simulink model "system_IIR_bank_decoder_AWGN"  (Simulink 8.3)
settings: Solver=ode45  StartTime=0.0  StopTime=10  RelTol=1e-3
undefined symbols (not defined in the file or in its folder): dfilt, fdesignblkfcn, gcbh
libraries: dsparch4 x7, commutil2 x2, commchan3 x1
settings Model: Creator=Vasilis  LastModifiedBy=Vasilis
settings DataIOCC: SignalLoggingSaveFormat=Dataset
settings DebuggingCC: UnderspecifiedInitializationDetection=Simplified  StateNameClashWarn=none
settings GRTTargetCC: CombineOutputUpdateFcns=on  GRTInterface=off

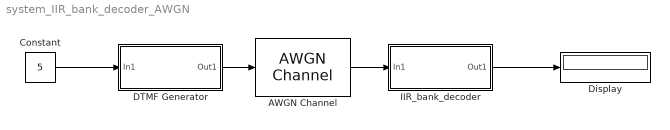
== system system_IIR_bank_decoder_AWGN ==
  AWGN Channel : commchan3/AWGN Channel  InputProcessing=Columns as channels (frame based)  seed=67  noiseMode="Signal to noise ratio  (SNR)"  EbNodB=10  EsNodB=10  SNRdB=0  bitsPerSym=1  Ps=1  Tsym=1  variance=1
  Constant : Constant  Value=5
  DTMF Generator : Subsystem
  Display : Display
  IIR_bank_decoder : Subsystem
  wires:
  DTMF Generator/1(Out1) -> AWGN Channel/1
  IIR_bank_decoder/1(Out1) -> Display/1
  Constant/1 -> DTMF Generator/1(In1)
  AWGN Channel/1 -> IIR_bank_decoder/1(In1)

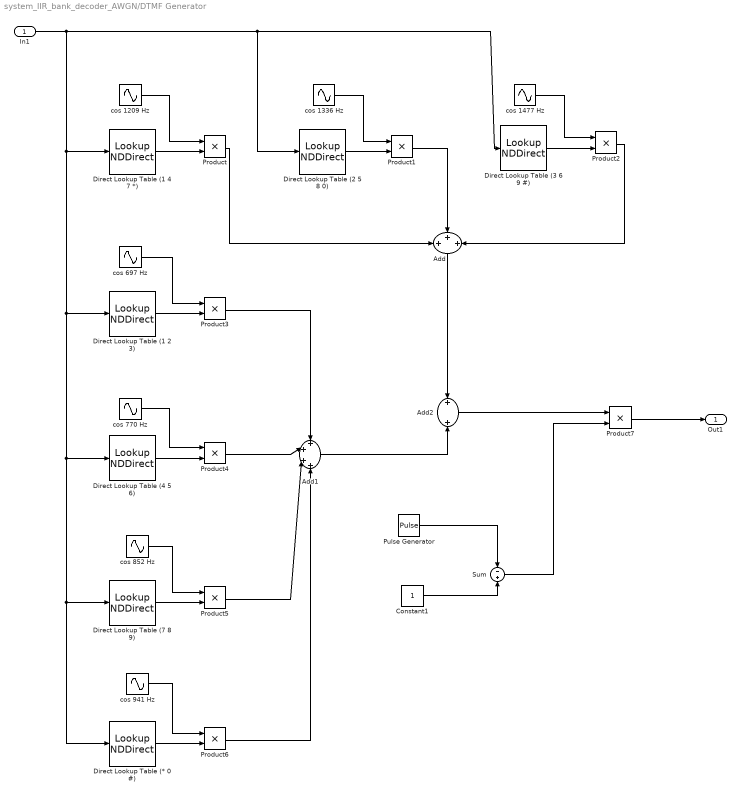
== system system_IIR_bank_decoder_AWGN/DTMF Generator ==
  In1 : Inport
  Add : Sum  Inputs=+++
  Add1 : Sum  Inputs=++++
  Add2 : Sum
  Constant1 : Constant
  Direct Lookup Table (* 0 #) : LookupNDDirect  NumberOfTableDimensions=1  Table=[1 0 0 0 0 0 0 0 0 0 1 1]
  Direct Lookup Table (1 2 3) : LookupNDDirect  NumberOfTableDimensions=1  Table=[0 1 1 1 0 0 0 0 0 0 0 0]
  Direct Lookup Table (1 4 7 *) : LookupNDDirect  NumberOfTableDimensions=1  Table=[0 1 0 0 1 0 0 1 0 0 1 0]
  Direct Lookup Table (2 5 8 0) : LookupNDDirect  NumberOfTableDimensions=1  Table=[1 0 1 0 0 1 0 0 1 0 0 0]
  Direct Lookup Table (3 6 9 #) : LookupNDDirect  NumberOfTableDimensions=1  Table=[0 0 0 1 0 0 1 0 0 1 0 1]
  Direct Lookup Table (4 5 6) : LookupNDDirect  NumberOfTableDimensions=1  Table=[0 0 0 0 1 1 1 0 0 0 0 0]
  Direct Lookup Table (7 8 9) : LookupNDDirect  NumberOfTableDimensions=1  Table=[0 0 0 0 0 0 0 1 1 1 0 0]
  Product{,1..7} (8 alike) : Product  RndMeth=Zero
  Pulse Generator : DiscretePulseGenerator  Period=480  PulseWidth=160  PhaseDelay=320  SampleTime=1/8000
  Sum : Sum  Inputs=-|+
  cos 1209 Hz : Sin  Frequency=7596  Phase=pi/2  SampleTime=1/8000
  cos 1336 Hz : Sin  Frequency=8394  Phase=pi/2  SampleTime=1/8000
  cos 1477 Hz : Sin  Frequency=9280  Phase=pi/2  SampleTime=1/8000
  cos 697 Hz : Sin  Frequency=4379  Phase=pi/2  SampleTime=1/8000
  cos 770 Hz : Sin  Frequency=4838  Phase=pi/2  SampleTime=1/8000
  cos 852 Hz : Sin  Frequency=5353  Phase=pi/2  SampleTime=1/8000
  cos 941 Hz : Sin  Frequency=5912  Phase=pi/2  SampleTime=1/8000
  Out1 : Outport
  wires:
  Direct Lookup Table (1 4 7 *)/1 -> Product/2
  In1/1 -> Direct Lookup Table (2 5 8 0)/1, Direct Lookup Table (3 6 9 #)/1, Direct Lookup Table (1 4 7 *)/1, Direct Lookup Table (1 2 3)/1, Direct Lookup Table (4 5 6)/1, Direct Lookup Table (7 8 9)/1, Direct Lookup Table (* 0 #)/1
  cos 1336 Hz/1 -> Product1/1
  Direct Lookup Table (2 5 8 0)/1 -> Product1/2
  cos 1477 Hz/1 -> Product2/1
  Direct Lookup Table (3 6 9 #)/1 -> Product2/2
  cos 697 Hz/1 -> Product3/1
  Direct Lookup Table (1 2 3)/1 -> Product3/2
  cos 770 Hz/1 -> Product4/1
  Direct Lookup Table (4 5 6)/1 -> Product4/2
  cos 852 Hz/1 -> Product5/1
  Direct Lookup Table (7 8 9)/1 -> Product5/2
  Product2/1 -> Add/3
  Product1/1 -> Add/2
  Product/1 -> Add/1
  Product3/1 -> Add1/1
  Product5/1 -> Add1/3
  Product4/1 -> Add1/2
  Add1/1 -> Add2/2
  Add/1 -> Add2/1
  cos 941 Hz/1 -> Product6/1
  Direct Lookup Table (* 0 #)/1 -> Product6/2
  Product6/1 -> Add1/4
  cos 1209 Hz/1 -> Product/1
  Constant1/1 -> Sum/2
  Pulse Generator/1 -> Sum/1
  Product7/1 -> Out1/1
  Add2/1 -> Product7/1
  Sum/1 -> Product7/2

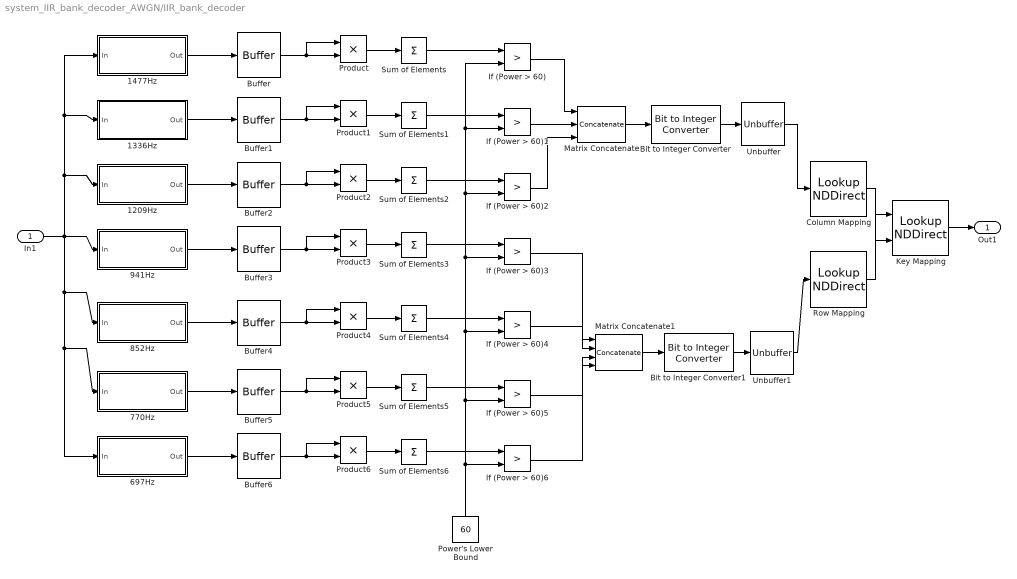
== system system_IIR_bank_decoder_AWGN/IIR_bank_decoder ==
  In1 : Inport
  1209Hz : Subsystem  DialogController=fdesignblkfcn  DialogControllerArgs=DataTag2  InitFcn=fdesignblkfcn(gcbh, {'InitFcn'});  mask(Bandpass Filter){}
      mask help: Design a bandpass filter
      settings: CopyFcn=fdesignblkfcn(gcbh, {'CopyFcn'});
      mask Help: helpview(mapfilelocation('dsp'), 'dspbandpassfilter');
      mask Display: disp('Bandpass');
  1336Hz : Subsystem  DialogController=fdesignblkfcn  DialogControllerArgs=DataTag5  InitFcn=fdesignblkfcn(gcbh, {'InitFcn'});  mask(Bandpass Filter){}
      mask help: Design a bandpass filter
      settings: CopyFcn=fdesignblkfcn(gcbh, {'CopyFcn'});
      mask Help: helpview(mapfilelocation('dsp'), 'dspbandpassfilter');
      mask Display: disp('Bandpass');
  1477Hz : Subsystem  DialogController=fdesignblkfcn  DialogControllerArgs=DataTag8  InitFcn=fdesignblkfcn(gcbh, {'InitFcn'});  mask(Bandpass Filter){}
      mask help: Design a bandpass filter
      settings: CopyFcn=fdesignblkfcn(gcbh, {'CopyFcn'});
      mask Help: helpview(mapfilelocation('dsp'), 'dspbandpassfilter');
      mask Display: disp('Bandpass');
  697Hz : Subsystem  DialogController=fdesignblkfcn  DialogControllerArgs=DataTag11  InitFcn=fdesignblkfcn(gcbh, {'InitFcn'});  mask(Bandpass Filter){}
      mask help: Design a bandpass filter
      settings: CopyFcn=fdesignblkfcn(gcbh, {'CopyFcn'});
      mask Help: helpview(mapfilelocation('dsp'), 'dspbandpassfilter');
      mask Display: disp('Bandpass');
  770Hz : Subsystem  DialogController=fdesignblkfcn  DialogControllerArgs=DataTag14  InitFcn=fdesignblkfcn(gcbh, {'InitFcn'});  mask(Bandpass Filter){}
      mask help: Design a bandpass filter
      settings: CopyFcn=fdesignblkfcn(gcbh, {'CopyFcn'});
      mask Help: helpview(mapfilelocation('dsp'), 'dspbandpassfilter');
      mask Display: disp('Bandpass');
  852Hz : Subsystem  DialogController=fdesignblkfcn  DialogControllerArgs=DataTag17  InitFcn=fdesignblkfcn(gcbh, {'InitFcn'});  mask(Bandpass Filter){}
      mask help: Design a bandpass filter
      settings: CopyFcn=fdesignblkfcn(gcbh, {'CopyFcn'});
      mask Help: helpview(mapfilelocation('dsp'), 'dspbandpassfilter');
      mask Display: disp('Bandpass');
  941Hz : Subsystem  DialogController=fdesignblkfcn  DialogControllerArgs=DataTag20  InitFcn=fdesignblkfcn(gcbh, {'InitFcn'});  mask(Bandpass Filter){}
      mask help: Design a bandpass filter
      settings: CopyFcn=fdesignblkfcn(gcbh, {'CopyFcn'});
      mask Help: helpview(mapfilelocation('dsp'), 'dspbandpassfilter');
      mask Display: disp('Bandpass');
  Bit to Integer Converter : commutil2/Bit to Integer Converter  nbits=3  bitOrder=MSB first  signedOutputValues=Unsigned  outDtype=Inherit via internal rule  outDtypeSigned=Inherit via internal rule
  Bit to Integer Converter1 : commutil2/Bit to Integer Converter  nbits=4  bitOrder=MSB first  signedOutputValues=Unsigned  outDtype=Inherit via internal rule  outDtypeSigned=Inherit via internal rule
  Buffer{,1..6} (7 alike) : Buffer  N=480  TreatMby1Signals=One channel
  Column Mapping : LookupNDDirect  NumberOfTableDimensions=1  Table=[0 1 2 0 3 0 0 0]
  If (Power > 60){,1..6} (7 alike) : RelationalOperator  Operator=>  OutDataTypeStr=boolean
  Key Mapping : LookupNDDirect  Table=[-1 -1 -1 -1;-1 1 2 3;-1 4 5 6;-1 7 8 9 ;-1 10 0 11]
  Matrix Concatenate : Concatenate  NumInputs=3  Mode=Multidimensional array
  Matrix Concatenate1 : Concatenate  NumInputs=4  Mode=Multidimensional array
  Power's Lower Bound : Constant  Value=60
  Product{,1..6} (7 alike) : Product  RndMeth=Zero
  Row Mapping : LookupNDDirect  NumberOfTableDimensions=1  Table=[0 1 2 0 3 0 0 4]
  Sum of Elements{,1..6} (7 alike) : Sum  Inputs=+
  Unbuffer : Unbuffer  SampleBasedProcessing=Same as frame based
  Unbuffer1 : Unbuffer  SampleBasedProcessing=Same as frame based
  Out1 : Outport
  wires:
  Product/1 -> Sum of Elements/1
  In1/1 -> 1477Hz/1(In), 1336Hz/1(In), 1209Hz/1(In), 852Hz/1(In), 697Hz/1(In), 770Hz/1(In), 941Hz/1(In)
  Product1/1 -> Sum of Elements1/1
  Product2/1 -> Sum of Elements2/1
  Product4/1 -> Sum of Elements4/1
  Product5/1 -> Sum of Elements5/1
  Product6/1 -> Sum of Elements6/1
  Sum of Elements/1 -> If (Power > 60)/1
  Sum of Elements1/1 -> If (Power > 60)1/1
  Sum of Elements2/1 -> If (Power > 60)2/1
  Sum of Elements4/1 -> If (Power > 60)4/1
  Sum of Elements5/1 -> If (Power > 60)5/1
  Sum of Elements6/1 -> If (Power > 60)6/1
  Power's Lower Bound/1 -> If (Power > 60)6/2, If (Power > 60)5/2, If (Power > 60)4/2, If (Power > 60)3/2, If (Power > 60)2/2, If (Power > 60)1/2, If (Power > 60)/2
  If (Power > 60)/1 -> Matrix Concatenate/1
  If (Power > 60)1/1 -> Matrix Concatenate/2
  If (Power > 60)2/1 -> Matrix Concatenate/3
  If (Power > 60)4/1 -> Matrix Concatenate1/2
  If (Power > 60)5/1 -> Matrix Concatenate1/3
  If (Power > 60)6/1 -> Matrix Concatenate1/4
  Matrix Concatenate/1 -> Bit to Integer Converter/1
  Matrix Concatenate1/1 -> Bit to Integer Converter1/1
  Product3/1 -> Sum of Elements3/1
  Sum of Elements3/1 -> If (Power > 60)3/1
  If (Power > 60)3/1 -> Matrix Concatenate1/1
  Column Mapping/1 -> Key Mapping/2
  Row Mapping/1 -> Key Mapping/1
  Key Mapping/1 -> Out1/1
  Unbuffer/1 -> Column Mapping/1
  Unbuffer1/1 -> Row Mapping/1
  Bit to Integer Converter1/1 -> Unbuffer1/1
  Bit to Integer Converter/1 -> Unbuffer/1
  Buffer/1 -> Product/1, Product/2
  Buffer1/1 -> Product1/1, Product1/2
  Buffer2/1 -> Product2/1, Product2/2
  Buffer3/1 -> Product3/1, Product3/2
  Buffer4/1 -> Product4/1, Product4/2
  Buffer5/1 -> Product5/1, Product5/2
  Buffer6/1 -> Product6/1, Product6/2
  1336Hz/1(Out) -> Buffer1/1
  1209Hz/1(Out) -> Buffer2/1
  941Hz/1(Out) -> Buffer3/1
  852Hz/1(Out) -> Buffer4/1
  770Hz/1(Out) -> Buffer5/1
  697Hz/1(Out) -> Buffer6/1
  1477Hz/1(Out) -> Buffer/1

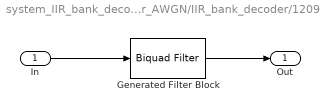
== system system_IIR_bank_decoder_AWGN/IIR_bank_decoder/1209Hz ==
  In : Inport
  Generated Filter Block : dsparch4/Biquad Filter  Tag=BlockMethodSubSystem  IIRFiltStruct=Direct form II  CoeffSource=Specify via dialog  BiQuadCoeffs=[0.011715658436785546 0 -0.011715658436785546 1 -1.1655017573289153 0.98641917045029659;0.0088825134997569995 0 -0.0088825134997569995 1 -1.1468268747980774 0.98630746856373164;0.0031436742187285769 0 -0.0031436742187285769 1 -1.1537994454093967 0.98223498363422623;0.017343223849340689 0 -0.017343223849340689 1 -1.1765831097499095 0.99691216940816552;0.0096918720050195219 0 -0.0096918720050195219 1 -1.1478984702170325 0.99687296779134338;0.011967241061030523 0 -0.011967241061030523 1 -1.1593718610728228 0.98333389809797711;0.0050685575395928613 0 -0.0050685575395928613 1 -1.1494424967958881 0.98326121040493009;0.015642365271632114 0 -0.015642365271632114 1 -1.1714720740726312 0.99112774721677632;0.61734335438585697 0 -0.61734335438585697 1 -1.1462827918644818 0.99102905804297059]  a0Flag=Warning  IC=0  ICnum=0  ICden=0  InputProcessing=Columns as channels (frame based)  denAccumFracLength=30  denProdOutputFracLength=30  secondMemoryFracLength=15  roundingMode=Floor  overflowMode=off  ScaleValues=[0.01099752574159257;1;1;1;1;1;1;1;1;1]  optimizeScaleValues=off  ScaleValueMode=Specify via input port (g)  scaleValueFracLength=14  FilterSource=Specify via dialog  dfiltObjectName=dfilt.df2tsos([1 0.3 0.4],[1 0.1 0.2])
  Out : Outport
  wires:
  In/1 -> Generated Filter Block/1
  Generated Filter Block/1 -> Out/1

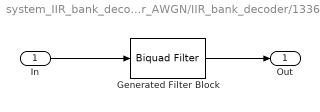
== system system_IIR_bank_decoder_AWGN/IIR_bank_decoder/1336Hz ==
  In : Inport
  Generated Filter Block : dsparch4/Biquad Filter  Tag=BlockMethodSubSystem  IIRFiltStruct=Direct form II  CoeffSource=Specify via dialog  BiQuadCoeffs=[0.011713430123475185 0 -0.011713430123475185 1 -0.9995232371900642 0.98638869255417028;0.0088952943484375911 0 -0.0088952943484375911 1 -0.97960610577415808 0.98629877383334708;0.0031574737728141257 0 -0.0031574737728141257 1 -0.98753771648865596 0.98220951994676453;0.017322139353942577 0 -0.017322139353942577 1 -1.0100840659278791 0.99690386096422723;0.0097226383823835454 0 -0.0097226383823835454 1 -0.9794619122617878 0.99687230338997335;0.011960265309811178 0 -0.011960265309811178 1 -0.99335206293477007 0.98330285709593601;0.0050883418582539563 0 -0.0050883418582539563 1 -0.98276515482096527 0.98324434485144319;0.015639369786377179 0 -0.015639369786377179 1 -1.0053283508921775 0.99110528101938222;0.57848309281864752 0 -0.57848309281864752 1 -0.97845193163444288 0.99102583646223741]  a0Flag=Warning  IC=0  ICnum=0  ICden=0  InputProcessing=Columns as channels (frame based)  denAccumFracLength=30  denProdOutputFracLength=30  secondMemoryFracLength=15  roundingMode=Floor  overflowMode=off  ScaleValues=[0.011762500891203136;1;1;1;1;1;1;1;1;1]  optimizeScaleValues=off  ScaleValueMode=Specify via input port (g)  scaleValueFracLength=14  FilterSource=Specify via dialog  dfiltObjectName=dfilt.df2tsos([1 0.3 0.4],[1 0.1 0.2])
  Out : Outport
  wires:
  In/1 -> Generated Filter Block/1
  Generated Filter Block/1 -> Out/1

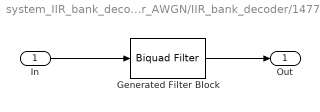
== system system_IIR_bank_decoder_AWGN/IIR_bank_decoder/1477Hz ==
  In : Inport
  Generated Filter Block : dsparch4/Biquad Filter  Tag=BlockMethodSubSystem  IIRFiltStruct=Direct form II  CoeffSource=Specify via dialog  BiQuadCoeffs=[0.011710837200687696 0 -0.011710837200687696 1 -0.80369052672120378 0.98635850606228215;0.0089080105864101002 0 -0.0089080105864101002 1 -0.78262094820308792 0.98629015080497306;0.0031672412018396881 0 -0.0031672412018396881 1 -0.79152882593879559 0.98218429228022663;0.01736076003755025 0 -0.01736076003755025 1 -0.81354529479121629 0.99689563238204293;0.0097177583520067553 0 -0.0097177583520067553 1 -0.78112714329091659 0.99687164214284452;0.011970708285959567 0 -0.011970708285959567 1 -0.79754544456707377 0.98327210975776713;0.0051035874736469478 0 -0.0051035874736469478 1 -0.78634837996143636 0.98322762970845712;0.015648712348332806 0 -0.015648712348332806 1 -0.80924278288880425 0.99108303060624992;0.54665795970879905 0 -0.54665795970879905 1 -0.78080176049205519 0.99102263706919835]  a0Flag=Warning  IC=0  ICnum=0  ICden=0  InputProcessing=Columns as channels (frame based)  denAccumFracLength=30  denProdOutputFracLength=30  secondMemoryFracLength=15  roundingMode=Floor  overflowMode=off  ScaleValues=[0.012476090590347143;1;1;1;1;1;1;1;1;1]  optimizeScaleValues=off  ScaleValueMode=Specify via input port (g)  scaleValueFracLength=14  FilterSource=Specify via dialog  dfiltObjectName=dfilt.df2tsos([1 0.3 0.4],[1 0.1 0.2])
  Out : Outport
  wires:
  In/1 -> Generated Filter Block/1
  Generated Filter Block/1 -> Out/1

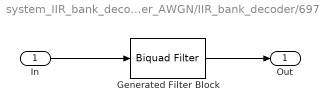
== system system_IIR_bank_decoder_AWGN/IIR_bank_decoder/697Hz ==
  In : Inport
  Generated Filter Block : dsparch4/Biquad Filter  Tag=BlockMethodSubSystem  IIRFiltStruct=Direct form II  CoeffSource=Specify via dialog  BiQuadCoeffs=[0.01393524053966029 0 -0.01393524053966029 1 -1.7059628142217351 0.98958852449003043;0.0079667606875477286 0 -0.0079667606875477286 1 -1.6914742497497404 0.98935143443269724;0.0097364126504748839 0 -0.0097364126504748839 1 -1.697672576693209 0.9841484152585056;0.002363601032442781 0 -0.002363601032442781 1 -1.6906525525294254 0.98397576600236036;0.017114677946963166 0 -0.017114677946963166 1 -1.7147187945080984 0.99776493640911978;0.0073826345817771645 0 -0.0073826345817771645 1 -1.6967372259304476 0.99770088754774122;0.015054106375185653 0 -0.015054106375185653 1 -1.7016170763686977 0.9864167935270608;0.010557842028326764 0 -0.010557842028326764 1 -1.690470390019609 0.98618043704742664;0.0088059425123732486 0 -0.0088059425123732486 1 -1.6943904346014227 0.98293787066329186;0.0046941483209824286 0 -0.0046941483209824286 1 -1.6919937602091606 0.98287474735520464;0.015837527835282687 0 -0.015837527835282687 1 -1.710426526154007 0.99345480986521673;0.97049875352683634 0 -0.97049875352683634 1 -1.6936089074502951 0.99328058100514072]  a0Flag=Warning  IC=0  ICnum=0  ICden=0  InputProcessing=Columns as channels (frame based)  denAccumFracLength=30  denProdOutputFracLength=30  secondMemoryFracLength=15  roundingMode=Floor  overflowMode=off  ScaleValues=[0.0053587470952647662;1;1;1;1;1;1;1;1;1;1;1;1]  optimizeScaleValues=off  ScaleValueMode=Specify via input port (g)  scaleValueFracLength=14  FilterSource=Specify via dialog  dfiltObjectName=dfilt.df2tsos([1 0.3 0.4],[1 0.1 0.2])
  Out : Outport
  wires:
  In/1 -> Generated Filter Block/1
  Generated Filter Block/1 -> Out/1

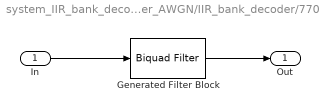
== system system_IIR_bank_decoder_AWGN/IIR_bank_decoder/770Hz ==
  In : Inport
  Generated Filter Block : dsparch4/Biquad Filter  Tag=BlockMethodSubSystem  IIRFiltStruct=Direct form II  CoeffSource=Specify via dialog  BiQuadCoeffs=[0.011724354640191059 0 -0.011724354640191059 1 -1.6406923024413462 0.98657395808501458;0.0088210413839329878 0 -0.0088210413839329878 1 -1.6275917380724894 0.98635143477002452;0.0030841280056484056 0 -0.0030841280056484056 1 -1.6308233951498026 0.98236418094107569;0.017297437400211668 0 -0.017297437400211668 1 -1.6526473655202087 0.99695437200512593;0.0096165387616449945 0 -0.0096165387616449945 1 -1.632689102844844 0.99687628911125148;0.011970253109740432 0 -0.011970253109740432 1 -1.6351672581895711 0.98349149379320611;0.0049765671540481851 0 -0.0049765671540481851 1 -1.6281852358942652 0.9833466828455204;0.015630353295319172 0 -0.015630353295319172 1 -1.6467520813117766 0.99124186158330607;0.88678407155490724 0 -0.88678407155490724 1 -1.6291461105190448 0.99104527601899184]  a0Flag=Warning  IC=0  ICnum=0  ICden=0  InputProcessing=Columns as channels (frame based)  denAccumFracLength=30  denProdOutputFracLength=30  secondMemoryFracLength=15  roundingMode=Floor  overflowMode=off  ScaleValues=[0.0075700455370004503;1;1;1;1;1;1;1;1;1]  optimizeScaleValues=off  ScaleValueMode=Specify via input port (g)  scaleValueFracLength=14  FilterSource=Specify via dialog  dfiltObjectName=dfilt.df2tsos([1 0.3 0.4],[1 0.1 0.2])
  Out : Outport
  wires:
  In/1 -> Generated Filter Block/1
  Generated Filter Block/1 -> Out/1

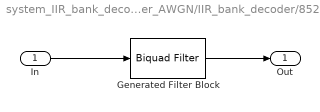
== system system_IIR_bank_decoder_AWGN/IIR_bank_decoder/852Hz ==
  In : Inport
  Generated Filter Block : dsparch4/Biquad Filter  Tag=BlockMethodSubSystem  IIRFiltStruct=Direct form II  CoeffSource=Specify via dialog  BiQuadCoeffs=[0.011721395855334433 0 -0.011721395855334433 1 -1.565183188118024 0.98653578246944462;0.0088367847006527653 0 -0.0088367847006527653 1 -1.5509110856985449 0.98634062239100773;0.0030965022713139723 0 -0.0030965022713139723 1 -1.5548774234377158 0.98233233697554145;0.01734002333129131 0 -0.01734002333129131 1 -1.5770901761350353 0.99694396245742434;0.0096191389912847289 0 -0.0096191389912847289 1 -1.5552917849778676 0.9968754784999232;0.011976298828046038 0 -0.011976298828046038 1 -1.5594924218113122 0.98345263396507399;0.0049975718307958845 0 -0.0049975718307958845 1 -1.55189158249124 0.98332563226238179;0.015637725152397135 0 -0.015637725152397135 1 -1.5712845120394725 0.99121371485200394;0.81188687850415786 0 -0.81188687850415786 1 -1.552082369571181 0.99104129932731189]  a0Flag=Warning  IC=0  ICnum=0  ICden=0  InputProcessing=Columns as channels (frame based)  denAccumFracLength=30  denProdOutputFracLength=30  secondMemoryFracLength=15  roundingMode=Floor  overflowMode=off  ScaleValues=[0.0082918604703149327;1;1;1;1;1;1;1;1;1]  optimizeScaleValues=off  ScaleValueMode=Specify via input port (g)  scaleValueFracLength=14  FilterSource=Specify via dialog  dfiltObjectName=dfilt.df2tsos([1 0.3 0.4],[1 0.1 0.2])
  Out : Outport
  wires:
  In/1 -> Generated Filter Block/1
  Generated Filter Block/1 -> Out/1

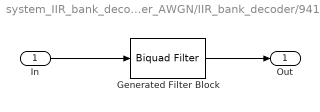
== system system_IIR_bank_decoder_AWGN/IIR_bank_decoder/941Hz ==
  In : Inport
  Generated Filter Block : dsparch4/Biquad Filter  Tag=BlockMethodSubSystem  IIRFiltStruct=Direct form II  CoeffSource=Specify via dialog  BiQuadCoeffs=[0.011720924904005305 0 -0.011720924904005305 1 -1.475902813978309 0.98650054769924289;0.0088490019430045915 0 -0.0088490019430045915 1 -1.4604202983332328 0.98633062442507147;0.003119861279445608 0 -0.003119861279445608 1 -1.4651698156578024 0.98230293404404334;0.017247374459336398 0 -0.017247374459336398 1 -1.4876960419644361 0.99693435540279585;0.0096864988818034115 0 -0.0096864988818034115 1 -1.4640006094037883 0.99687472527467569;0.011947024158331064 0 -0.011947024158331064 1 -1.4700589576401772 0.98341676274132772;0.0050257347014900037 0 -0.0050257347014900037 1 -1.461818349470233 0.98330618562036387;0.015620731882434589 0 -0.015620731882434589 1 -1.482018563890263 0.99118773782887648;0.74690907172149612 0 -0.74690907172149612 1 -1.461168914068329 0.99103761520940092]  a0Flag=Warning  IC=0  ICnum=0  ICden=0  InputProcessing=Columns as channels (frame based)  denAccumFracLength=30  denProdOutputFracLength=30  secondMemoryFracLength=15  roundingMode=Floor  overflowMode=off  ScaleValues=[0.0090353285999899297;1;1;1;1;1;1;1;1;1]  optimizeScaleValues=off  ScaleValueMode=Specify via input port (g)  scaleValueFracLength=14  FilterSource=Specify via dialog  dfiltObjectName=dfilt.df2tsos([1 0.3 0.4],[1 0.1 0.2])
  Out : Outport
  wires:
  In/1 -> Generated Filter Block/1
  Generated Filter Block/1 -> Out/1
